simulink model "experiment2017b"  (R2017b)
settings: Solver=VariableStepAuto  StartTime=0.0  StopTime=10  FixedStep=td  RelTol=1e-5  EnableMultiTasking=on
values from neighbouring files (symbols this model uses):
  A = lstm1_getContinuousA(I_zz,c_alpha_fl,c_alpha_fr,c_alpha_rl,c_alpha_rr,l_f,l_r,m,v)    [run_experiment.m]
  Ad = sysd.a    [run_experiment.m]
  B = lstm1_getContinuousB(I_zz,c_alpha_fl,c_alpha_fr,c_alpha_rl,c_alpha_rr,l_f,l_r,m,v)    [run_experiment.m]
  Bd = sysd.b    [run_experiment.m]
  C = [C_psi_dot;C_ay]    [run_experiment.m]
  Cd = sysd.c    [run_experiment.m]
  D = [D_psi_dot;D_ay]    [run_experiment.m]
  Dd = sysd.d    [run_experiment.m]
  P0 = zeros(2,2)    [run_experiment.m]
  Q_real = diag([0.005,0.001])    [run_experiment.m]
  Qd_kf = Qd_real*noise_factor    [run_experiment.m]
  Qd_real = Q_real*td^2    [run_experiment.m]
  qm_real = [0.01;0.01]*0    [run_experiment.m]
  qmd_real = qm_real*td    [run_experiment.m]
  R_real = diag([0.05,0.03])    [run_experiment.m]
  Rd_kf = Rd_real    [run_experiment.m]
  Rd_real = R_real    [run_experiment.m]
  rm_real = [0.1;0.1]*0    [run_experiment.m]
  rmd_real = rm_real    [run_experiment.m]
  Simulated_Sensor_Offset = [0;                                 0]    [run_experiment.m]
  td = 0.001    [run_experiment.m]
  x0 = lstm1_buildX(psi_dot,beta)    [run_experiment.m]
  x0_hat = x0    [run_experiment.m]
settings Model: Creator=S2J2XWE  LastModifiedBy=Ossig
settings DataIOCC: LimitDataPoints=on
settings OptimizationCC: LifeSpan=inf
settings DebuggingCC: AllowSymbolicDim=off  SFUnexpectedBacktrackingDiag=warning  SFNoUnconditionalDefaultTransitionDiag=warning  SFExecutionAtInitializationDiag=none
settings ModelReferenceCC: PropagateSignalLabelsOutOfModel=off
settings CodeAppCC: StateflowObjectComments=on
settings GRTTargetCC: TargetLangStandard=C89/C90 (ANSI)
settings ConfigComp: CovMetricSettings=dw  CovHtmlReporting=on  CovSaveCumulativeToWorkspaceVar=on  CovSaveSingleToWorkspaceVar=on  CovExternalEMLEnable=off

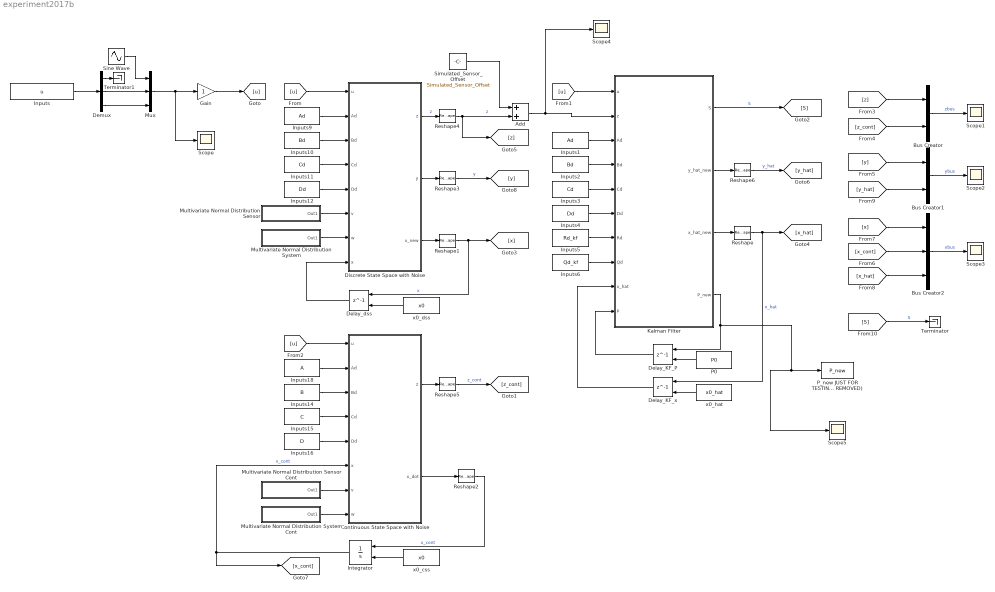
== system experiment2017b ==
  Add : Sum
  Bus Creator : BusCreator  Inputs=2
  Bus Creator1 : BusCreator  Inputs=2
  Bus Creator2 : BusCreator  Inputs=3
  Continuous State Space with Noise : MATLAB Function  TreatAsAtomicUnit=on
  Delay_KF_P : Delay  DelayLength=1  InitialConditionSource=Input port  SampleTime=td
      settings: InputPortMap=u0,p4
  Delay_KF_x : Delay  DelayLength=1  InitialConditionSource=Input port  SampleTime=td
      settings: InputPortMap=u0,p4
  Delay_dss : Delay  DelayLength=1  InitialConditionSource=Input port  SampleTime=td
      settings: InputPortMap=u0,p4
  Demux : Demux  Outputs=3
  Discrete State Space with Noise : MATLAB Function  TreatAsAtomicUnit=on
  Gain : Gain
  Inputs : Constant  Value=u  VectorParams1D=off  SampleTime=td
  Inputs1 : Constant  Value=Ad  SampleTime=td
  Inputs10 : Constant  Value=Bd  SampleTime=td
  Inputs11 : Constant  Value=Cd  SampleTime=td
  Inputs12 : Constant  Value=Dd  SampleTime=td
  Inputs14 : Constant  Value=B  SampleTime=td
  Inputs15 : Constant  Value=C  SampleTime=td
  Inputs16 : Constant  Value=D  SampleTime=td
  Inputs18 : Constant  Value=A  SampleTime=td
  Inputs2 : Constant  Value=Bd  SampleTime=td
  Inputs3 : Constant  Value=Cd  SampleTime=td
  Inputs4 : Constant  Value=Dd  SampleTime=td
  Inputs5 : Constant  Value=Rd_kf  SampleTime=td
  Inputs6 : Constant  Value=Qd_kf  SampleTime=td
  Inputs9 : Constant  Value=Ad  SampleTime=td
  Integrator : Integrator  InitialConditionSource=external
  Kalman Filter : MATLAB Function  TreatAsAtomicUnit=on
  Multivariate Normal Distribution Sensor : Subsystem  mask(Multivariate Normal Distribution){m=rmd_real, P=Rd_real, seed=[0;1], td=td}
      mask prompts: m "Mean"; P "Covariance matrix"; seed "Initial seed"; td "Sample time"
      mask help:
      | Output a multivariate normally (Gaussian) distributed random signal.
      |
      | (like described by Peter Junglas (http://www.peter-junglas.de/fh/vorlesungen/skripte/kalman.pdf))
      mask init:
      | [C,res]= sqrtm(P);
      mask Help: http://www.peter-junglas.de/fh/vorlesungen/skripte/kalman.pdf
      mask Display: disp('N(m,P)')
  Multivariate Normal Distribution Sensor Cont : Subsystem  mask(Multivariate Normal Distribution){m=rm_real, P=R_real, seed=[0;1], td=td}
      mask prompts: m "Mean"; P "Covariance matrix"; seed "Initial seed"; td "Sample time"
      mask help:
      | Output a multivariate normally (Gaussian) distributed random signal.
      |
      | (like described by Peter Junglas (http://www.peter-junglas.de/fh/vorlesungen/skripte/kalman.pdf))
      mask init:
      | [C,res]= sqrtm(P);
      mask Help: http://www.peter-junglas.de/fh/vorlesungen/skripte/kalman.pdf
      mask Display: disp('N(m,P)')
  Multivariate Normal Distribution System : Subsystem  mask(Multivariate Normal Distribution){m=qmd_real, P=Qd_real, seed=[5;10], td=td}
      mask prompts: m "Mean"; P "Covariance matrix"; seed "Initial seed"; td "Sample time"
      mask help:
      | Output a multivariate normally (Gaussian) distributed random signal.
      |
      | (like described by Peter Junglas (http://www.peter-junglas.de/fh/vorlesungen/skripte/kalman.pdf))
      mask init:
      | [C,res]= sqrtm(P);
      mask Help: http://www.peter-junglas.de/fh/vorlesungen/skripte/kalman.pdf
      mask Display: disp('N(m,P)')
  Multivariate Normal Distribution System Cont : Subsystem  mask(Multivariate Normal Distribution){m=qm_real, P=Q_real, seed=[0;1], td=td}
      mask prompts: m "Mean"; P "Covariance matrix"; seed "Initial seed"; td "Sample time"
      mask help:
      | Output a multivariate normally (Gaussian) distributed random signal.
      |
      | (like described by Peter Junglas (http://www.peter-junglas.de/fh/vorlesungen/skripte/kalman.pdf))
      mask init:
      | [C,res]= sqrtm(P);
      mask Help: http://www.peter-junglas.de/fh/vorlesungen/skripte/kalman.pdf
      mask Display: disp('N(m,P)')
  Mux : Mux  Inputs=3
  P0 : Constant  Value=P0  VectorParams1D=off  SampleTime=td
  P_new JUST FOR TESTING (CAN BE REMOVED) : ToWorkspace  VariableName=P_new  SaveFormat=Timeseries  SampleTime=-1
  Reshape{,1..6} (7 alike) : Reshape  OutputDimensionality=Column vector (2-D)
  Scope{,1..5} (6 alike) : Scope
  Simulated_Sensor_Offset : Constant  Value=Simulated_Sensor_Offset
  Sine Wave : Sin  Amplitude=deg2rad(5)  SampleTime=0
  Terminator : Terminator
  Terminator1 : Terminator
  x0_css : Constant  Value=x0  VectorParams1D=off  SampleTime=td
  x0_dss : Constant  Value=x0  VectorParams1D=off  SampleTime=td
  x0_hat : Constant  Value=x0_hat  VectorParams1D=off  SampleTime=td
  wires:
  Inputs1/1 -> Kalman Filter/3(Ad)
  Inputs2/1 -> Kalman Filter/4(Bd)
  Inputs3/1 -> Kalman Filter/5(Cd)
  Inputs4/1 -> Kalman Filter/6(Dd)
  Inputs5/1 -> Kalman Filter/7(Rd)
  Inputs6/1 -> Kalman Filter/8(Qd)
  x0_hat/1 -> Delay_KF_x/2
  P0/1 -> Delay_KF_P/2
  Kalman Filter/4(P_new) -> P_new JUST FOR TESTING (CAN BE REMOVED)/1, Scope5/1, Delay_KF_P/1
  Delay_KF_P/1 -> Kalman Filter/10(P)
  Kalman Filter/3(x_hat_new) -> Reshape/1
  Delay_KF_x/1 -> Kalman Filter/9(x_hat)
  Reshape/1 -> Delay_KF_x/1, [x_hat]  "x_hat"
  Inputs9/1 -> Discrete State Space with Noise/2(Ad)
  Inputs10/1 -> Discrete State Space with Noise/3(Bd)
  Inputs11/1 -> Discrete State Space with Noise/4(Cd)
  Inputs12/1 -> Discrete State Space with Noise/5(Dd)
  Delay_dss/1 -> Discrete State Space with Noise/8(x)
  x0_dss/1 -> Delay_dss/2
  Discrete State Space with Noise/3(x_new) -> Reshape1/1
  Reshape1/1 -> Delay_dss/1, [x]  "x"
  Multivariate Normal Distribution Sensor/1(Out1) -> Discrete State Space with Noise/6(v)
  Multivariate Normal Distribution System/1(Out1) -> Discrete State Space with Noise/7(w)
  Inputs18/1 -> Continuous State Space with Noise/2(Ad)
  Inputs14/1 -> Continuous State Space with Noise/3(Bd)
  Inputs15/1 -> Continuous State Space with Noise/4(Cd)
  Inputs16/1 -> Continuous State Space with Noise/5(Dd)
  Integrator/1 -> Continuous State Space with Noise/6(x), [x_cont]  "x_cont"
  x0_css/1 -> Integrator/2
  Continuous State Space with Noise/2(x_dot) -> Reshape2/1
  Reshape2/1 -> Integrator/1  "x_cont"
  Multivariate Normal Distribution Sensor Cont/1(Out1) -> Continuous State Space with Noise/7(v)
  Multivariate Normal Distribution System Cont/1(Out1) -> Continuous State Space with Noise/8(w)
  Continuous State Space with Noise/1(z) -> Reshape5/1
  Gain/1 -> [u]
  [u] -> Discrete State Space with Noise/1(u)
  [u] -> Kalman Filter/1(u)
  [u] -> Continuous State Space with Noise/1(u)
  Kalman Filter/1(S) -> [S]  "S"
  Kalman Filter/2(y_hat_new) -> Reshape6/1
  [z_cont] -> Bus Creator/2
  [z] -> Bus Creator/1
  [y] -> Bus Creator1/1
  Bus Creator/1 -> Scope1/1  "zbus"
  Discrete State Space with Noise/1(z) -> Reshape4/1  "z"
  Discrete State Space with Noise/2(y) -> Reshape3/1
  [y_hat] -> Bus Creator1/2
  Bus Creator1/1 -> Scope2/1  "ybus"
  [x] -> Bus Creator2/1
  [x_cont] -> Bus Creator2/2
  [x_hat] -> Bus Creator2/3
  Bus Creator2/1 -> Scope3/1  "xbus"
  [S] -> Terminator/1  "S"
  Reshape3/1 -> [y]  "y"
  Reshape4/1 -> Add/2, [z]  "z"
  Reshape5/1 -> [z_cont]  "z_cont"
  Reshape6/1 -> [y_hat]  "y_hat"
  Add/1 -> Kalman Filter/2(z), Scope4/1
  Simulated_Sensor_Offset/1 -> Add/1
  Sine Wave/1 -> Mux/1
  Inputs/1 -> Demux/1
  Demux/3 -> Mux/3
  Demux/2 -> Mux/2
  Demux/1 -> Terminator1/1
  Mux/1 -> Gain/1, Scope/1

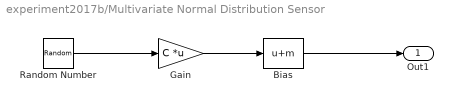
== system experiment2017b/Multivariate Normal Distribution Sensor ==
  Bias : Bias  Bias=m
  Gain : Gain  Gain=C  Multiplication=Matrix(K*u)
  Random Number : RandomNumber  Seed=seed  SampleTime=td  VectorParams1D=off
  Out1 : Outport  VectorParamsAs1DForOutWhenUnconnected=off
  wires:
  Bias/1 -> Out1/1
  Gain/1 -> Bias/1
  Random Number/1 -> Gain/1

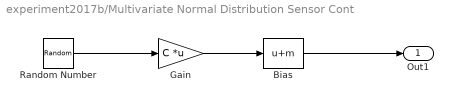
== system experiment2017b/Multivariate Normal Distribution Sensor Cont ==
  Bias : Bias  Bias=m
  Gain : Gain  Gain=C  Multiplication=Matrix(K*u)
  Random Number : RandomNumber  Seed=seed  SampleTime=td  VectorParams1D=off
  Out1 : Outport  VectorParamsAs1DForOutWhenUnconnected=off
  wires:
  Bias/1 -> Out1/1
  Gain/1 -> Bias/1
  Random Number/1 -> Gain/1

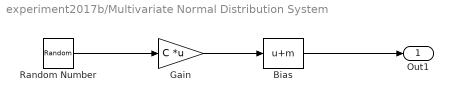
== system experiment2017b/Multivariate Normal Distribution System ==
  Bias : Bias  Bias=m
  Gain : Gain  Gain=C  Multiplication=Matrix(K*u)
  Random Number : RandomNumber  Seed=seed  SampleTime=td  VectorParams1D=off
  Out1 : Outport  VectorParamsAs1DForOutWhenUnconnected=off
  wires:
  Random Number/1 -> Gain/1
  Gain/1 -> Bias/1
  Bias/1 -> Out1/1

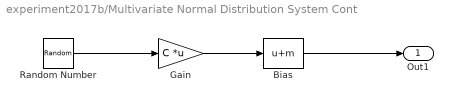
== system experiment2017b/Multivariate Normal Distribution System Cont ==
  Bias : Bias  Bias=m
  Gain : Gain  Gain=C  Multiplication=Matrix(K*u)
  Random Number : RandomNumber  Seed=seed  SampleTime=td  VectorParams1D=off
  Out1 : Outport  VectorParamsAs1DForOutWhenUnconnected=off
  wires:
  Random Number/1 -> Gain/1
  Gain/1 -> Bias/1
  Bias/1 -> Out1/1

== matlab function experiment2017b/Discrete State Space with Noise ==
  data: z output; y output; x_new output; u input; Ad input; Bd input; Cd input; Dd input; v input; w input; x input
function [z,y,x_new]  = fcn(u,Ad,Bd,Cd,Dd,v,w,x)
%%%%%%%%%%%%%%%%%%%%%%%%%%%%%%%%%%%%%%%%%%%%%%%%%%%%%%%%%%%%%%%%%%%%%%%%%%
% Author:       Daniel Ossig
% Date:         26.07.2018
%
% Description:
%
% MATLAB Vers.: 2017a
%
%%%%%%%%%%%%%%%%%%%%%%%%%%%%%%%%%%%%%%%%%%%%%%%%%%%%%%%%%%%%%%%%%%%%%%%%%%
%#codegen


x_new = Ad*x+Bd*u+w;
y     = Cd*x+Dd*u;
z     = y+v;

== matlab function experiment2017b/Kalman Filter ==
  data: S output; y_hat_new output; u input; z input; Ad input; Bd input; Cd input; Dd input; Rd input; Qd input; x_hat input; P input; x_hat_new output; P_new output
function [S,y_hat_new,x_hat_new,P_new] = fcn(u,z,Ad,Bd,Cd,Dd,Rd,Qd,x_hat,P)
%%%%%%%%%%%%%%%%%%%%%%%%%%%%%%%%%%%%%%%%%%%%%%%%%%%%%%%%%%%%%%%%%%%%%%%%%%
% Author:       Daniel Ossig
% Date:         26.07.2018
%
% Description:
%
% MATLAB Vers.: 2017a
%
%%%%%%%%%%%%%%%%%%%%%%%%%%%%%%%%%%%%%%%%%%%%%%%%%%%%%%%%%%%%%%%%%%%%%%%%%%
%#codegen

n=size(Ad,1);

% predict
x_hat_pred = Ad*x_hat+Bd*u;
P_pred     = Ad*P*Ad'+Qd;

% update
v          = z - Cd*x_hat_pred-Dd*u;
S          = Rd + Cd*P_pred*Cd';

K          = P*Cd'/S;
x_hat_new  = x_hat_pred + K*v;
P_new      = (eye(n)-K*Cd)*P_pred;

y_hat_new  = Cd*x_hat_new+Dd*u;

== matlab function experiment2017b/Continuous State Space with Noise ==
  data: z output; u input; Ad input; Bd input; Cd input; Dd input; x input; v input; x_dot output; w input
function [z,x_dot]  = fcn(u,Ad,Bd,Cd,Dd,x,v,w)
%%%%%%%%%%%%%%%%%%%%%%%%%%%%%%%%%%%%%%%%%%%%%%%%%%%%%%%%%%%%%%%%%%%%%%%%%%
% Author:       Daniel Ossig
% Date:         26.07.2018
%
% Description:
%
% MATLAB Vers.: 2017a
%
%%%%%%%%%%%%%%%%%%%%%%%%%%%%%%%%%%%%%%%%%%%%%%%%%%%%%%%%%%%%%%%%%%%%%%%%%%
%#codegen


x_dot = Ad*x+Bd*u+w;
z     = Cd*x+Dd*u+v;
